simulink model "Assignment2_3"  (R2021a)
settings: Solver=VariableStepAuto  StartTime=0.0  StopTime=10  RelTol=1e-3
settings Model: Creator=mstra  LastModifiedBy=Luca
settings SolverCC: AlgebraicLoopSolver=TrustRegion
settings DebuggingCC: SFMachineParentedDataDiag=warning

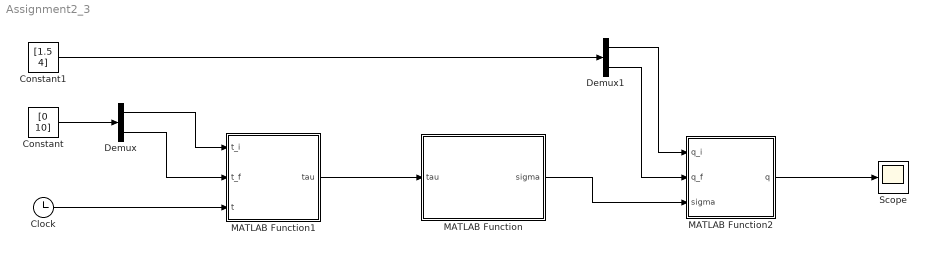
== system Assignment2_3 ==
  Clock : Clock
  Constant : Constant  Value=[0 10]
  Constant1 : Constant  Value=[1.5 4]
  Demux : Demux  Outputs=2
  Demux1 : Demux  Outputs=2
  MATLAB Function : MATLAB Function  TreatAsAtomicUnit=on
  MATLAB Function1 : MATLAB Function  TreatAsAtomicUnit=on
  MATLAB Function2 : MATLAB Function  TreatAsAtomicUnit=on
  Scope : Scope
  wires:
  MATLAB Function/1(sigma) -> MATLAB Function2/3(sigma)
  MATLAB Function1/1(tau) -> MATLAB Function/1(tau)
  Clock/1 -> MATLAB Function1/3(t)
  Constant/1 -> Demux/1
  Demux/1 -> MATLAB Function1/1(t_i)
  Demux/2 -> MATLAB Function1/2(t_f)
  MATLAB Function2/1(q) -> Scope/1
  Constant1/1 -> Demux1/1
  Demux1/1 -> MATLAB Function2/1(q_i)
  Demux1/2 -> MATLAB Function2/2(q_f)

== matlab function Assignment2_3/MATLAB Function1 ==
  data: t_i input; tau output; t_f input; t input
function tau = t2tau(t_i,t_f,t)
% Compute the value of tau. 
% INPUT: 
% -	t_i: initial time 
% -	t_f: final time 
% - t: symbolic time variable
% OUTPUT:
% - tau 
%

T = t_f - t_i;
tau = (t - t_i)/T;

== matlab function Assignment2_3/MATLAB Function ==
  data: sigma output; tau input
function sigma  = sim_poly_trajD5(tau)
% Compute sigma
% INPUT: 
% - tau 
% OUTPUT: 
% - sigma 

sigma = 10*tau^3 - 15*tau^4 + 6*tau^5;

end

== matlab function Assignment2_3/MATLAB Function2 ==
  data: q_i input; q output; q_f input; sigma input
function q = fcn(q_i,q_f,sigma)
% compute position at time t
% INPUT: 
% -	q_i: initial value (i.e., value at t_i) 
% -	q_f: final value (i.e., value at time t_f) 
% - sigma
% OUTPUT:
% - q: position at time t

h = q_f - q_i;
q = q_i + h * sigma;
